simulink model "chart_dbg_demo"  (R2021a)
settings: Solver=VariableStepAuto  StartTime=0.0  StopTime=10.0  RelTol=1e-3
undefined symbols (not defined in the file): sigbuilder_block
settings Model: Creator=DELL  LastModifiedBy=DELL

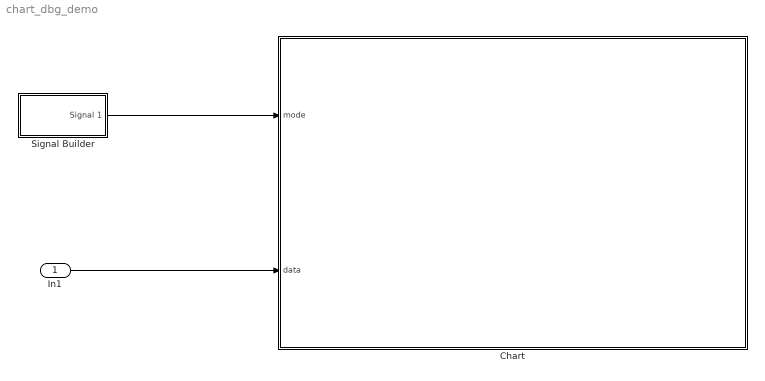
== system chart_dbg_demo ==
  In1 : Inport
  Chart : Stateflow chart  TreatAsAtomicUnit=on
  Signal Builder : Subsystem  Tag=STV Subsys  LoadFcn=sigbuilder_block('load');  StartFcn=sigbuilder_block('start');  StopFcn=sigbuilder_block('stop');  ClipboardFcn=sigbuilder_block('clipboard');  mask(Sigbuilder block){tuvar=[0:10]}
      mask help: Simulink:masks:SigbuilderBlock_MD
      mask init:
      | if ~strcmp(get_param(bdroot(gcbh),'SimulationStatus'),'stopped') tuvar = sigbuilder_block('maskInit'); end
      settings: CopyFcn=sigbuilder_block('copy');  DeleteFcn=sigbuilder_block('delete');  ModelCloseFcn=sigbuilder_block('modelClose');  PreSaveFcn=sigbuilder_block('preSave');  PauseFcn=sigbuilder_block('pause');  ContinueFcn=sigbuilder_block('continue');  NameChangeFcn=sigbuilder_block('namechange');  OpenFcn=sigbuilder_block('open',[437.6 199.2 550.4 400 ]);  CloseFcn=sigbuilder_block('close');
      mask Display: plot(0, 0, 100, 100,[2, 2, 32, 32, 2], [68, 8, 8, 68, 68],[32, 2], [38, 38], [32, 19, 2],[53, 60, 44], [32, 17, 17, 2],[16, 16, 31, 31]);txt = getActiveGroup(gcbh);text(2, 100, txt,'verticalAlignment', 'top');
  wires:
  Signal Builder/1(Signal 1) -> Chart/1(mode)
  In1/1 -> Chart/2(data)

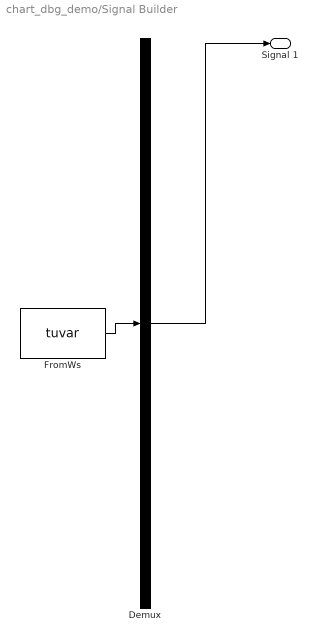
== system chart_dbg_demo/Signal Builder ==
  Demux : Demux  Tag=STV Demux  Outputs=1
      settings: DisplayOption=none
  FromWs : FromWorkspace  Tag=STV FromWs  VariableName=tuvar
      SigBuilderData=|
      | common.afterFinalStr = 'Extrapolate'
      | common.sampleTime = 0
      | dataSet.timeRange = [0 10]
      | dataSet.name = 'Group 1'
      | sbobj.Groups.Name = 'Group 1'
      | sbobj.Groups.Signals.Name = 'Signal 1'
      | sbobj.Groups.Signals.XData = [0 4 4 8 8 10]
      | sbobj.Groups.Signals.YData = [1 1 2 2 1 1]
  Signal 1 : Outport  Tag=STV Outport
  wires:
  Demux/1 -> Signal 1/1
  FromWs/1 -> Demux/1

== stateflow chart chart_dbg_demo/Chart ==
  state fffff
    en:
    sfdbg('fff en')
    du:
    sfdbg('fff du')
    ex:
    sfdbg('fff ex')
    state SETPOINT_TYPE_IDLE
      en:
      sfdbg('idle en')
      du:
      sfdbg('idle du')
      ex:
      sfdbg('idle ex')
    state SETPOINT_TYPE_TAKEOFF
      en:
      sfdbg('take en')
      du:
      sfdbg('take du')
      ssss()
      ex:
      sfdbg('take,ex')
    state SETPOINT_TYPE_TAKEOFF1
      en:
      sfdbg('take1 en')
      du:
      sfdbg('take1 du')
      ex:
      sfdbg('take,ex')
    fffff -> (junction 9) : [hasChanged(mode)]{sfdbg('to inner')}
    (default) -> (junction 9)
    (junction 9) -> SETPOINT_TYPE_IDLE [order 1] : [mode ==1]
    (junction 9) -> (junction 4) [order 2]
    SETPOINT_TYPE_IDLE -> SETPOINT_TYPE_TAKEOFF : [mode ==2||after(1,sec)]{sfdbg('to take')}
    SETPOINT_TYPE_TAKEOFF -> SETPOINT_TYPE_IDLE : [mode == 1]{sfdbg('to idle')}
    (junction 4) -> SETPOINT_TYPE_TAKEOFF [order 1] : [mode==2]
    (junction 4) -> SETPOINT_TYPE_TAKEOFF1 [order 2]
  (default) -> fffff
  data: mode input; data input
